simulink model "e01_MtrCtrl_VarGain"  (R2024a)
settings: Solver=FixedStepDiscrete  StartTime=0.0  StopTime=1  FixedStep=mSim.dTime  MaxStep=Define.sModelSampleTime  RelTol=7.1420e-05
undefined symbols (not defined in the file): CnstMde, E01CCG, E01PCG, E01SCG
settings Model: Creator=user  LastModifiedBy=admin
settings SolverCC: MaxConsecutiveZCs=10000  ZeroCrossAlgorithm=Adaptive  AlgebraicLoopSolver=TrustRegion
settings DataIOCC: SaveOutput=off  DSMLogging=off  InspectSignalLogs=on  SaveTime=off  SignalLoggingName=logsout_Validator
settings OptimizationCC: BlockReduction=off  DefaultParameterBehavior=Inlined  UseDivisionForNetSlopeComputation=UseDivisionForReciprocalsOfIntegersOnly  GainParamInheritBuiltInType=on  UseFloatMulNetSlope=on  DefaultUnderspecifiedDataType=single  InlineInvariantSignals=on  BitwiseOrLogicalOp=Logical operator  PassReuseOutputArgsAs=Individual arguments  EfficientFloat2IntCast=on  LifeSpan=Inf  OptimizeBlockOrder=speed  DifferentSizesBufferReuse=on  EfficientTunableParamExpr=on
settings DebuggingCC: SignalInfNanChecking=error  SignalRangeChecking=error  ReadBeforeWriteMsg=EnableAllAsError  WriteAfterWriteMsg=EnableAllAsError  WriteAfterReadMsg=EnableAllAsError  AlgebraicLoopMsg=error  ArtificialAlgebraicLoopMsg=error  SaveWithDisabledLinksMsg=error  SaveWithParameterizedLinksMsg=error  BlockPriorityViolationMsg=error  SolverPrmCheckMsg=error  InheritedTsInSrcMsg=error  SingleTaskRateTransMsg=error  TasksWithSamePriorityMsg=error  SigSpecEnsureSampleTimeMsg=error  CheckMatrixSingularityMsg=error  IntegerOverflowMsg=error  ParameterUnderflowMsg=error  ParameterPrecisionLossMsg=error  ParameterTunabilityLossMsg=error  UnderSpecifiedDataTypeMsg=error  UnnecessaryDatatypeConvMsg=warning  VectorMatrixConversionMsg=error  SignalLabelMismatchMsg=error  UnconnectedInputMsg=error  UnconnectedOutputMsg=error  UnconnectedLineMsg=error  SFcnCompatibilityMsg=error  UniqueDataStoreMsg=error  BusObjectLabelMismatch=error  RootOutportRequireBusObject=error  AssertControl=DisableAll  ModelReferenceIOMismatchMessage=error  UnknownTsInhSupMsg=error  ModelReferenceDataLoggingMessage=error  ModelReferenceSymbolNameMessage=none  StateNameClashWarn=warning  StrictBusMsg=ErrorOnBusTreatedAsVector  NonBusSignalsTreatedAsBus=error  SFInvalidInputDataAccessInChartInitDiag=error  SFTransitionOutsideNaturalParentDiag=error  SFUnreachableExecutionPathDiag=error  SFUndirectedBroadcastEventsDiag=error  SFTransitionActionBeforeConditionDiag=error  SFTemporalDelaySmallerThanSampleTimeDiag=error  SFSelfTransitionDiag=error  SFExecutionAtInitializationDiag=error  IntegerSaturationMsg=error  UnitsInconsistencyMsg=none  VariantConditionMismatch=error
settings HardwareCC: ProdBitPerChar=16  ProdBitPerInt=16  ProdBitPerPointer=32  ProdBitPerSizeT=32  ProdBitPerPtrDiffT=32  ProdLargestAtomicInteger=Integer  ProdLargestAtomicFloat=None  ProdWordSize=16  ProdLongLongMode=on  ProdHWDeviceType=Texas Instruments->C2000
settings ModelReferenceCC: EnableRefExpFcnMdlSchedulingChecks=on  ModelReferenceNumInstancesAllowed=Single
settings SFSimCC: SimUseLocalCustomCode=off  CompileTimeRecursionLimit=0  EnableRuntimeRecursion=off  MATLABDynamicMemAlloc=off  CustomCodeUndefinedFunction=UseInterfaceOnly
settings RTWCC: Description=Embedded Coder  SystemTargetFile=ert.tlc  GenCodeOnly=on  TemplateMakefile=ert_default_tmf  GenerateReport=on  RTWUseLocalCustomCode=off  BuildConfiguration=Faster Runs  IncludeHyperlinkInReport=on  LaunchReport=on  GenerateTraceInfo=on  GenerateTraceReport=on  GenerateTraceReportSl=on  GenerateTraceReportSf=on  GenerateWebview=on  GenerateCodeMetricsReport=on  GenerateCodeReplacementReport=on  GPUComputeCapability=3.5  DLArmComputeVersion=19.05
settings CodeAppCC: ForceParamTrailComments=on  IgnoreCustomStorageClasses=off  MATLABFcnDesc=on  MangleLength=4  CustomSymbolStrGlobalVar=GvE01$N$M  CustomSymbolStrType=StrE01$N$M  CustomSymbolStrFcn=$N$M$F  CustomSymbolStrMacro=$N$M  DefineNamingRule=UpperCase  ParamNamingRule=UpperCase  SimulinkBlockComments=off  MATLABSourceComments=on  EnableCustomComments=on  ReqsInCode=on
settings ERTTargetCC: UtilityFuncGeneration=Shared location  MultiwordLength=2048  IncludeMdlTerminateFcn=off  CombineSignalStateStructs=on  SuppressErrorStatus=on  SupportAbsoluteTime=off  SupportNonFinite=off  ParenthesesLevel=Maximum  CastingMode=Standards  GenerateSharedConstants=off  InlinedParameterPlacement=NonHierarchical  ERTSrcFileBannerTemplate=t_code_template.cgt  ERTHdrFileBannerTemplate=t_code_template.cgt  ERTDataSrcFileTemplate=t_code_template.cgt  ERTDataHdrFileTemplate=t_code_template.cgt  ERTCustomFileTemplate=example_file_process.tlc  ERTFilePackagingFormat=CompactWithDataFile  PreserveExpressionOrder=on  SuppressUnreachableDefaultCases=off  EnableSignedLeftShifts=off  EnableSignedRightShifts=off  IndentStyle=Allman  IndentSize=4
settings ConfigComp: CovSaveName=coveragedata  CovMetricSettings=we  CovEnableCumulative=off  CovSaveCumulativeToWorkspaceVar=on  CovSaveSingleToWorkspaceVar=on  CovOutputDir=sldv_output/$ModelName$\sldv_covoutput  PSVerificationMode=BugFinder  PSModelRefIgnoreList=[]  PSEnableModelRefIgnoreList=off  PSModelRefMinMaxVerif=CheckAndConstrain  PSAutoStubLUT=on  DVModelCoverageObjectives=MCDC  DVTestSuiteOptimization=CombinedObjectives (Nonlinear Extended)  DVRebuildModelRepresentation=Always
settings SimscapeCC: SimscapeNormalizeSystem=off

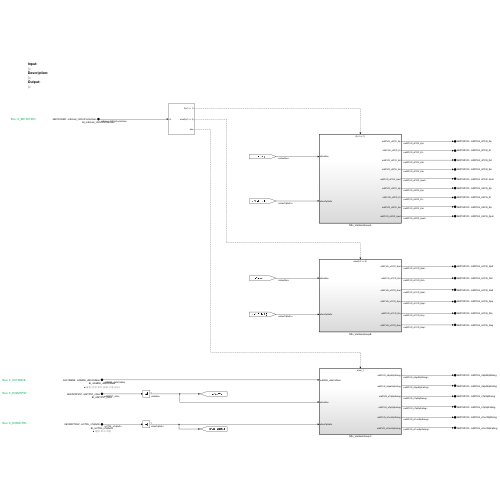
[thumbnail: Simulink's stored preview of the top-level diagram]
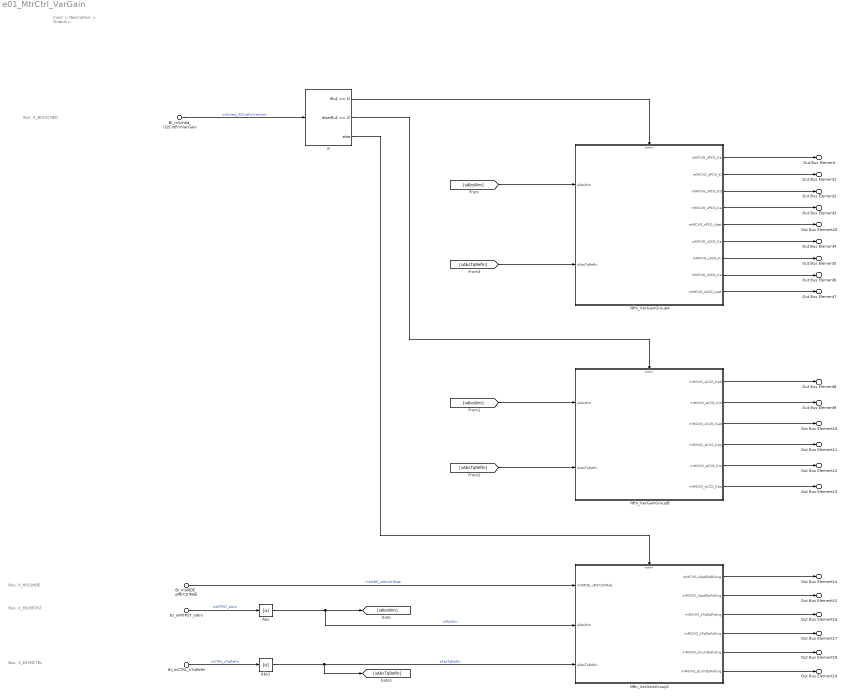
== system e01_MtrCtrl_VarGain ==
  note: Bus: X_H01SMDE
  note: Input:
      | ▷
      | Description:
      | ▷
      | Output:
      | ▷
  note: Bus: X_E02MTPST
  note: Bus: X_E03MCTRL
  note: Bus: X_B01SCHED
  BI_mSMDE_uMtrCtrlMde : Inport  Description=■ 설명: 운영 모드 (모터 구동 모드)  PortName=bH01SMDE  Element=mSMDE_uMtrCtrlMde
      settings: AttributesFormatString=%<Description>
  BI_mMTPST_sWm : Inport  Description=■ 설명: 기계 각속도 (Wm = 12000 * 2pi/60)  Port=2  PortName=bE02MTPSTZ  Element=mMTPST_sWm
      settings: AttributesFormatString=%<Description>
  BI_mSched_i32CntForVarGain : Inport  Description=■ 설명: 가변게인 스케쥴 카운터  Port=3  PortName=bB01SCHED  Element=mSched_i32CntForVarGain
  BI_mCTRL_sTqRefIn : Inport  Description=■ 설명: 토크 지령  Port=4  PortName=bE03MCTRLZ  Element=mCTRL_sTqRefIn
      settings: AttributesFormatString=%<Description>
  Abs : Abs  SaturateOnIntegerOverflow=off
  Abs1 : Abs  SaturateOnIntegerOverflow=off
  If : If  IfExpression=u1 == 1  ElseIfExpressions=u1 == 2
  Nftn_VarGainGroupA : Subsystem  TreatAsAtomicUnit=on
      settings: RTWFcnNameOpts=Use subsystem name
  Nftn_VarGainGroupB : Subsystem  TreatAsAtomicUnit=on
      settings: RTWFcnNameOpts=Use subsystem name
  Nftn_VarGainGroupC : Subsystem  TreatAsAtomicUnit=on
      settings: RTWFcnNameOpts=Use subsystem name
  Out Bus Element : Outport  Description=■ 설명: 위치 제어 게인 Kp  PortName=bE01MCVG  Element=mMCVG_sPCG_Kp
  Out Bus Element1 : Outport  Description=■ 설명: 위치 제어 게인 Ki  PortName=bE01MCVG  Element=mMCVG_sPCG_Ki
  Out Bus Element2 : Outport  Description=■ 설명: 위치 제어 게인 Kd  PortName=bE01MCVG  Element=mMCVG_sPCG_Kd
  Out Bus Element3 : Outport  Description=■ 설명: 위치 제어 게인 Ka  PortName=bE01MCVG  Element=mMCVG_sPCG_Ka
  Out Bus Element20 : Outport  Description=■ 설명: 가속도 게인  PortName=bE01MCVG  Element=mMCVG_sPCG_Apst
  Out Bus Element4 : Outport  Description=■ 설명: 속도 제어 게인 Kp  PortName=bE01MCVG  Element=mMCVG_sSCG_Kp
  Out Bus Element5 : Outport  Description=■ 설명: 속도 제어 게인 Ki  PortName=bE01MCVG  Element=mMCVG_sSCG_Ki
  Out Bus Element6 : Outport  Description=■ 설명: 속도 제어 게인 Ka  PortName=bE01MCVG  Element=mMCVG_sSCG_Ka
  Out Bus Element7 : Outport  Description=■ 설명: 속도 제어 게인 Apst  PortName=bE01MCVG  Element=mMCVG_sSCG_Apst
  Out Bus Element8 : Outport  Description=■ 설명: d축 전류 제어 게인 Kp  PortName=bE01MCVG  Element=mMCVG_sCCG_Kpd
  Out Bus Element9 : Outport  Description=■ 설명: d축 전류 제어 게인 Ki  PortName=bE01MCVG  Element=mMCVG_sCCG_Kid
  Out Bus Element10 : Outport  Description=■ 설명: d축 전류 제어 게인 Ka  PortName=bE01MCVG  Element=mMCVG_sCCG_Kad
  Out Bus Element11 : Outport  Description=■ 설명: q축 전류 제어 게인 Kp  PortName=bE01MCVG  Element=mMCVG_sCCG_Kpq
  Out Bus Element12 : Outport  Description=■ 설명: q축 전류 제어 게인 Ki  PortName=bE01MCVG  Element=mMCVG_sCCG_Kiq
  Out Bus Element13 : Outport  Description=■ 설명: q축 전류 제어 게인 Ka  PortName=bE01MCVG  Element=mMCVG_sCCG_Kaq
  Out Bus Element14 : Outport  Description=■ 설명: 속도 제어 지령 가속 기울기  PortName=bE01MCVG  Element=mMCVG_sSpdSlpRising
  Out Bus Element15 : Outport  Description=■ 설명: 속도 제어 지령 감속 기울기  PortName=bE01MCVG  Element=mMCVG_sSpdSlpFalling
  Out Bus Element16 : Outport  Description=■ 설명: 토크 제어 지령 가속 기울기  PortName=bE01MCVG  Element=mMCVG_sTqSlpRising
  Out Bus Element17 : Outport  Description=■ 설명: 토크 제어 지령 감속 기울기  PortName=bE01MCVG  Element=mMCVG_sTqSlpFalling
  Out Bus Element18 : Outport  Description=■ 설명: 전류 제어 지령 가속 기울기  PortName=bE01MCVG  Element=mMCVG_sCurrSlpRising
  Out Bus Element19 : Outport  Description=■ 설명: 전류 제어 지령 감속 기울기  PortName=bE01MCVG  Element=mMCVG_sCurrSlpFalling
  wires:
  BI_mSched_i32CntForVarGain/1 -> If/1  "mSched_i32CntForVarGain"
  If/1 -> Nftn_VarGainGroupA/Action
  If/2 -> Nftn_VarGainGroupB/Action
  If/3 -> Nftn_VarGainGroupC/Action
  BI_mMTPST_sWm/1 -> Abs/1  "mMTPST_sWm"
  [sAbsWm] -> Nftn_VarGainGroupA/1(sAbsWm)
  [sAbsWm] -> Nftn_VarGainGroupB/1(sAbsWm)
  BI_mCTRL_sTqRefIn/1 -> Abs1/1  "mCTRL_sTqRefIn"
  [sAbsTqRefIn] -> Nftn_VarGainGroupB/2(sAbsTqRefIn)
  [sAbsTqRefIn] -> Nftn_VarGainGroupA/2(sAbsTqRefIn)
  Nftn_VarGainGroupA/1(mMCVG_sPCG_Kp) -> Out Bus Element/1
  Nftn_VarGainGroupA/2(mMCVG_sPCG_Ki) -> Out Bus Element1/1
  Nftn_VarGainGroupA/3(mMCVG_sPCG_Kd) -> Out Bus Element2/1
  Nftn_VarGainGroupA/4(mMCVG_sPCG_Ka) -> Out Bus Element3/1
  Nftn_VarGainGroupA/6(mMCVG_sSCG_Kp) -> Out Bus Element4/1
  Nftn_VarGainGroupA/7(mMCVG_sSCG_Ki) -> Out Bus Element5/1
  Nftn_VarGainGroupA/8(mMCVG_sSCG_Ka) -> Out Bus Element6/1
  Nftn_VarGainGroupA/9(mMCVG_sSCG_Apst) -> Out Bus Element7/1
  Nftn_VarGainGroupB/1(mMCVG_sCCG_Kpd) -> Out Bus Element8/1
  Nftn_VarGainGroupB/2(mMCVG_sCCG_Kid) -> Out Bus Element9/1
  Nftn_VarGainGroupB/3(mMCVG_sCCG_Kad) -> Out Bus Element10/1
  Nftn_VarGainGroupB/4(mMCVG_sCCG_Kpq) -> Out Bus Element11/1
  Nftn_VarGainGroupB/5(mMCVG_sCCG_Kiq) -> Out Bus Element12/1
  Nftn_VarGainGroupB/6(mMCVG_sCCG_Kaq) -> Out Bus Element13/1
  Nftn_VarGainGroupC/1(mMCVG_sSpdSlpRising) -> Out Bus Element14/1
  Nftn_VarGainGroupC/2(mMCVG_sSpdSlpFalling) -> Out Bus Element15/1
  Nftn_VarGainGroupC/3(mMCVG_sTqSlpRising) -> Out Bus Element16/1
  Nftn_VarGainGroupC/4(mMCVG_sTqSlpFalling) -> Out Bus Element17/1
  Nftn_VarGainGroupC/5(mMCVG_sCurrSlpRising) -> Out Bus Element18/1
  Nftn_VarGainGroupC/6(mMCVG_sCurrSlpFalling) -> Out Bus Element19/1
  Nftn_VarGainGroupA/5(mMCVG_sPCG_Apst) -> Out Bus Element20/1
  BI_mSMDE_uMtrCtrlMde/1 -> Nftn_VarGainGroupC/1(mSMDE_uMtrCtrlMde)  "mSMDE_uMtrCtrlMde"
  Abs/1 -> Nftn_VarGainGroupC/2(sAbsWm), [sAbsWm]  "sAbsWm"
  Abs1/1 -> [sAbsTqRefIn], Nftn_VarGainGroupC/3(sAbsTqRefIn)  "sAbsTqRefIn"

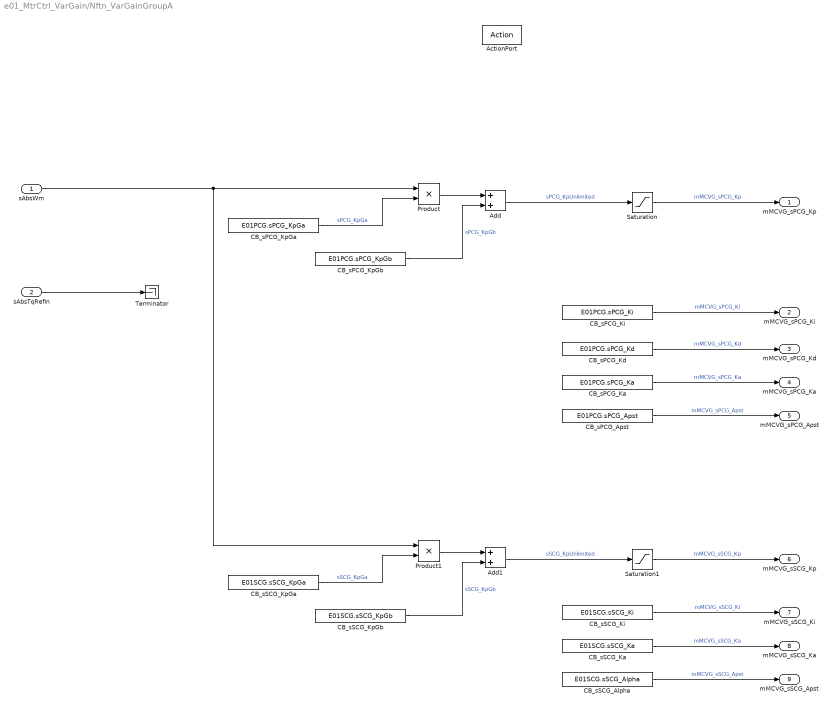
== system e01_MtrCtrl_VarGain/Nftn_VarGainGroupA ==
  sAbsWm : Inport
  sAbsTqRefIn : Inport  Port=2
  ActionPort : ActionPort  ActionPortLabel=if(u1 == 1)
  Add : Sum
  Add1 : Sum
  CB_sPCG_Apst : Constant  Value=E01PCG.sPCG_Apst
  CB_sPCG_Ka : Constant  Value=E01PCG.sPCG_Ka
  CB_sPCG_Kd : Constant  Value=E01PCG.sPCG_Kd
  CB_sPCG_Ki : Constant  Value=E01PCG.sPCG_Ki
  CB_sPCG_KpGa : Constant  Value=E01PCG.sPCG_KpGa
  CB_sPCG_KpGb : Constant  Value=E01PCG.sPCG_KpGb
  CB_sSCG_Alpha : Constant  Value=E01SCG.sSCG_Alpha
  CB_sSCG_Ka : Constant  Value=E01SCG.sSCG_Ka
  CB_sSCG_Ki : Constant  Value=E01SCG.sSCG_Ki
  CB_sSCG_KpGa : Constant  Value=E01SCG.sSCG_KpGa
  CB_sSCG_KpGb : Constant  Value=E01SCG.sSCG_KpGb
  Product : Product
  Product1 : Product
  Saturation : Saturate  UpperLimit=E01PCG.sPCG_KpMax  LowerLimit=E01PCG.sPCG_KpMin
  Saturation1 : Saturate  UpperLimit=E01SCG.sSCG_KpMax  LowerLimit=E01SCG.sSCG_KpMin
  Terminator : Terminator
  mMCVG_sPCG_Kp : Outport
  mMCVG_sPCG_Ki : Outport  Port=2
  mMCVG_sPCG_Kd : Outport  Port=3
  mMCVG_sPCG_Ka : Outport  Port=4
  mMCVG_sPCG_Apst : Outport  Port=5
  mMCVG_sSCG_Kp : Outport  Port=6
  mMCVG_sSCG_Ki : Outport  Port=7
  mMCVG_sSCG_Ka : Outport  Port=8
  mMCVG_sSCG_Apst : Outport  Port=9
  wires:
  Saturation/1 -> mMCVG_sPCG_Kp/1  "mMCVG_sPCG_Kp"
  Add/1 -> Saturation/1  "sPCG_KpUnlimited"
  CB_sPCG_KpGa/1 -> Product/2  "sPCG_KpGa"
  Product/1 -> Add/1
  CB_sPCG_KpGb/1 -> Add/2  "sPCG_KpGb"
  CB_sPCG_Ki/1 -> mMCVG_sPCG_Ki/1  "mMCVG_sPCG_Ki"
  CB_sPCG_Kd/1 -> mMCVG_sPCG_Kd/1  "mMCVG_sPCG_Kd"
  CB_sPCG_Ka/1 -> mMCVG_sPCG_Ka/1  "mMCVG_sPCG_Ka"
  CB_sPCG_Apst/1 -> mMCVG_sPCG_Apst/1  "mMCVG_sPCG_Apst"
  CB_sSCG_Ki/1 -> mMCVG_sSCG_Ki/1  "mMCVG_sSCG_Ki"
  CB_sSCG_Alpha/1 -> mMCVG_sSCG_Apst/1  "mMCVG_sSCG_Apst"
  CB_sSCG_Ka/1 -> mMCVG_sSCG_Ka/1  "mMCVG_sSCG_Ka"
  CB_sSCG_KpGb/1 -> Add1/2  "sSCG_KpGb"
  Product1/1 -> Add1/1
  CB_sSCG_KpGa/1 -> Product1/2  "sSCG_KpGa"
  Add1/1 -> Saturation1/1  "sSCG_KpUnlimited"
  Saturation1/1 -> mMCVG_sSCG_Kp/1  "mMCVG_sSCG_Kp"
  sAbsWm/1 -> Product/1, Product1/1
  sAbsTqRefIn/1 -> Terminator/1

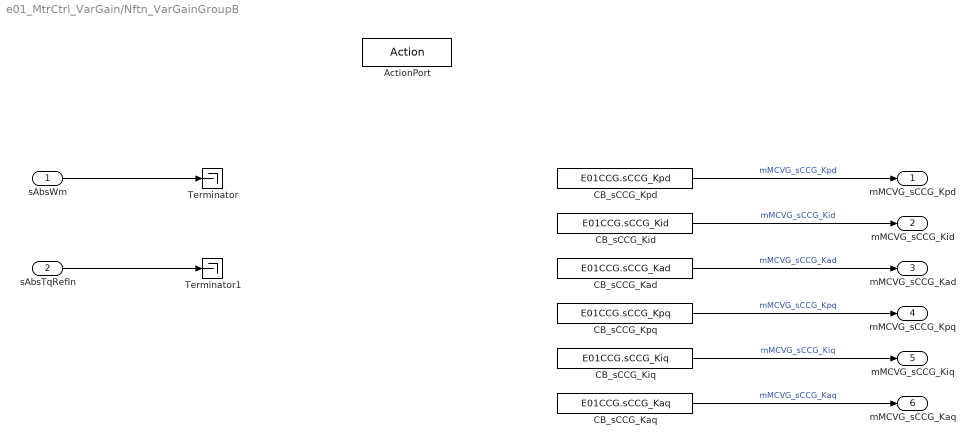
== system e01_MtrCtrl_VarGain/Nftn_VarGainGroupB ==
  sAbsWm : Inport
  sAbsTqRefIn : Inport  Port=2
  ActionPort : ActionPort  ActionPortLabel=elseif(u1 == 2)
  CB_sCCG_Kad : Constant  Value=E01CCG.sCCG_Kad
  CB_sCCG_Kaq : Constant  Value=E01CCG.sCCG_Kaq
  CB_sCCG_Kid : Constant  Value=E01CCG.sCCG_Kid
  CB_sCCG_Kiq : Constant  Value=E01CCG.sCCG_Kiq
  CB_sCCG_Kpd : Constant  Value=E01CCG.sCCG_Kpd
  CB_sCCG_Kpq : Constant  Value=E01CCG.sCCG_Kpq
  Terminator : Terminator
  Terminator1 : Terminator
  mMCVG_sCCG_Kpd : Outport
  mMCVG_sCCG_Kid : Outport  Port=2
  mMCVG_sCCG_Kad : Outport  Port=3
  mMCVG_sCCG_Kpq : Outport  Port=4
  mMCVG_sCCG_Kiq : Outport  Port=5
  mMCVG_sCCG_Kaq : Outport  Port=6
  wires:
  sAbsWm/1 -> Terminator/1
  sAbsTqRefIn/1 -> Terminator1/1
  CB_sCCG_Kpd/1 -> mMCVG_sCCG_Kpd/1  "mMCVG_sCCG_Kpd"
  CB_sCCG_Kid/1 -> mMCVG_sCCG_Kid/1  "mMCVG_sCCG_Kid"
  CB_sCCG_Kad/1 -> mMCVG_sCCG_Kad/1  "mMCVG_sCCG_Kad"
  CB_sCCG_Kpq/1 -> mMCVG_sCCG_Kpq/1  "mMCVG_sCCG_Kpq"
  CB_sCCG_Kiq/1 -> mMCVG_sCCG_Kiq/1  "mMCVG_sCCG_Kiq"
  CB_sCCG_Kaq/1 -> mMCVG_sCCG_Kaq/1  "mMCVG_sCCG_Kaq"

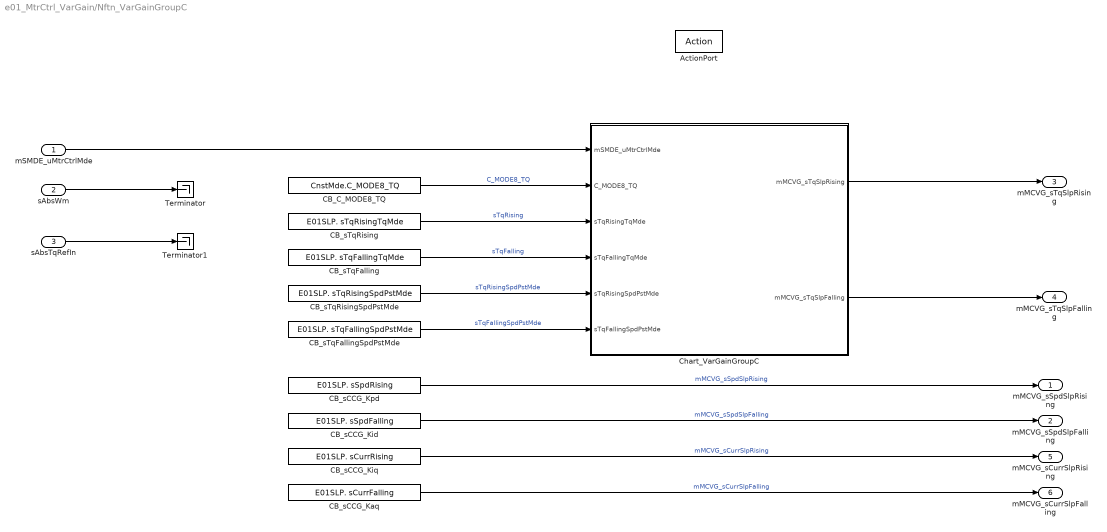
== system e01_MtrCtrl_VarGain/Nftn_VarGainGroupC ==
  mSMDE_uMtrCtrlMde : Inport
  sAbsWm : Inport  Port=2
  sAbsTqRefIn : Inport  Port=3
  ActionPort : ActionPort  ActionPortLabel=else
  CB_C_MODE8_TQ : Constant  Value=CnstMde.C_MODE8_TQ
  CB_sCCG_Kaq : Constant  Value=E01SLP. sCurrFalling
  CB_sCCG_Kid : Constant  Value=E01SLP. sSpdFalling
  CB_sCCG_Kiq : Constant  Value=E01SLP. sCurrRising
  CB_sCCG_Kpd : Constant  Value=E01SLP. sSpdRising
  CB_sTqFalling : Constant  Value=E01SLP. sTqFallingTqMde
  CB_sTqFallingSpdPstMde : Constant  Value=E01SLP. sTqFallingSpdPstMde
  CB_sTqRising : Constant  Value=E01SLP. sTqRisingTqMde
  CB_sTqRisingSpdPstMde : Constant  Value=E01SLP. sTqRisingSpdPstMde
  Chart_VarGainGroupC : Stateflow chart  TreatAsAtomicUnit=on
  Terminator : Terminator
  Terminator1 : Terminator
  mMCVG_sSpdSlpRising : Outport
  mMCVG_sSpdSlpFalling : Outport  Port=2
  mMCVG_sTqSlpRising : Outport  Port=3
  mMCVG_sTqSlpFalling : Outport  Port=4
  mMCVG_sCurrSlpRising : Outport  Port=5
  mMCVG_sCurrSlpFalling : Outport  Port=6
  wires:
  sAbsWm/1 -> Terminator/1
  sAbsTqRefIn/1 -> Terminator1/1
  CB_sCCG_Kiq/1 -> mMCVG_sCurrSlpRising/1  "mMCVG_sCurrSlpRising"
  CB_sCCG_Kaq/1 -> mMCVG_sCurrSlpFalling/1  "mMCVG_sCurrSlpFalling"
  CB_sCCG_Kpd/1 -> mMCVG_sSpdSlpRising/1  "mMCVG_sSpdSlpRising"
  Chart_VarGainGroupC/1(mMCVG_sTqSlpRising) -> mMCVG_sTqSlpRising/1
  CB_sCCG_Kid/1 -> mMCVG_sSpdSlpFalling/1  "mMCVG_sSpdSlpFalling"
  Chart_VarGainGroupC/2(mMCVG_sTqSlpFalling) -> mMCVG_sTqSlpFalling/1
  CB_sTqRising/1 -> Chart_VarGainGroupC/3(sTqRisingTqMde)  "sTqRising"
  CB_sTqFalling/1 -> Chart_VarGainGroupC/4(sTqFallingTqMde)  "sTqFalling"
  CB_sTqRisingSpdPstMde/1 -> Chart_VarGainGroupC/5(sTqRisingSpdPstMde)  "sTqRisingSpdPstMde"
  CB_sTqFallingSpdPstMde/1 -> Chart_VarGainGroupC/6(sTqFallingSpdPstMde)  "sTqFallingSpdPstMde"
  mSMDE_uMtrCtrlMde/1 -> Chart_VarGainGroupC/1(mSMDE_uMtrCtrlMde)
  CB_C_MODE8_TQ/1 -> Chart_VarGainGroupC/2(C_MODE8_TQ)  "C_MODE8_TQ"

== stateflow chart e01_MtrCtrl_VarGain/Nftn_VarGainGroupC/Chart_VarGainGroupC ==
  (default) -> (junction 15)
  (junction 15) -> (junction 16) [order 1] : [mSMDE_uMtrCtrlMde == C_MODE8_TQ]
  (junction 15) -> (junction 17) [order 2] : {
      | mMCVG_sTqSlpRising = sTqRisingSpdPstMde;
      | mMCVG_sTqSlpFalling = sTqFallingSpdPstMde;
      | }
  (junction 16) -> (junction 18) : {
      | mMCVG_sTqSlpRising = sTqRisingTqMde;
      | mMCVG_sTqSlpFalling = sTqFallingTqMde;
      | }
  (junction 18) -> (junction 17)
  (junction 17) -> (junction 19)
  data: mSMDE_uMtrCtrlMde input; C_MODE8_TQ input; mMCVG_sTqSlpRising output single; mMCVG_sTqSlpFalling output single; sTqRisingTqMde input; sTqFallingTqMde input; sTqRisingSpdPstMde input; sTqFallingSpdPstMde input
